simulink model "test"  (R2017b)
settings: Solver=FixedStepDiscrete  StartTime=0.0  StopTime=Inf  FixedStep=Ts  RelTol=1e-3
PreLoadFcn:
  | Ts = 0.01;
PostLoadFcn:
  | , if any(exist('dsrtsu_mdlpostloadfcn', 'file') == [2, 3, 6]), try dsrtsu_mdlpostloadfcn('Execute', bdroot); catch fprintf('Error in PostLoadFcn (dsrtsu_mdlpostloadfcn) for model "%s":\n %s\n', bdroot, lasterr); end, end,
libraries: rtican x19, simulink x9, rti1401lib_adc_type4 x3
(part 5 of 6)

== system test/Hardware ActValue/Suspension Motor RX ==
  N20_TPDO0 : rtican/RTICAN Receive (RX)   Reserved1=[]  Reserved2=[]  Reserved3=[]  Reserved4=[]  SfcnMessage=[]  Msg_Struct=[]  BoardTypeNo=[]  BoardNo=[]  ChannelNo=[]  Parameters=[]  DialogFcn=[]  UnitName=[]  Revision=[]  UnitValues=[]  DSProperties=struct('RTI',struct('Version',uint32(5),'BlockType',struct('isSLSource',uint8(1),'isSLSink',uint8(1),'isHWSource',uint8(0),'isHWSink',uint8(0),'isSetup',uint8(0),'isInline',uint8(1),'isNonInline',uint8(0),'isInterrupt',uint8(0),'isChannelwise',uint8(0)),'IOBoardType','RTICAN','UnitType','MESSAGE','Identifier','RX','DialogType','MSVC','BlockSet','RTICAN','SlaveProcessor','CAN'))  RTIBlockInterface=struct('OutputPortsWidth',int32([1 1 1 1 1 1 1]),'OutputPortsActive',[1 1 1 1 1 1 1],'OutputPortsName',{{'Controlword','Statusword','Modes_of_operation_display','Error_code',['RX status'],['RX time'],['RX delta time']}},'OutputPortsDataType',{{'SS_DOUBLE','SS_DOUBLE','SS_DOUBLE','SS_DOUBLE','SS_DOUBLE','SS_DOUBLE','SS_DOUBLE'}},'OutputPortsLabel',{{'Controlword','Statusword','Modes_of_operation_display','Error_code','','',''}},'OutputPortsLabelMode','ON','InputPortsWidth',int32(0),'InputPortsActive',0,'DialogFcn','rtican_message_interface_gui','BlockDisplay',{{'','center'}},'IconTransparency','on','ParameterTunableNames',{{}},'InitLevel',3,'BlockName',struct('Token',{{'N20_TPDO0'}}),'SampleTime',{{-1}},'TriggerPort',{{'none'}},'EnablePort',{{'none'}})  RTIBlockParameters=struct('BoardTypeNo',{{1,'OFF',[]}},'BoardNo',{{1,'ON',[1 16]}},'ChannelNo',{{1,'ON',[1 2]}},'Parameters',{{struct('DataFileSupport',struct('DataFileSelectedMaster',1,'DataFileSelectedLocal',1,'DataFileName','c:\users\user\desktop\ycm\rcp\can1_canopen.dbc|','DataFileDate',['16-7-2025 15:06:12'],'SelectedFile',['..\..\ycm\rcp\ycm_canopen_v1 .dbc'],'InterfaceFcn','rtican_dbc_file_parser'),'Options',struct('StatusSelected',1,'TimeSelected',1,'DeltaTimeSelected',1,'BytePortSelected',0,'MessageLengthSelected',0,'TriggerPort',struct('Selected',0,'TriggerType',0),'UserCoding',struct('Selected',0,'InterfaceFile','UserDecodingFile','FcnName','UserDecodeFcn','InportSelected',0,'InportWidth',1,'OutportSelected',0,'OutportWidth',1),'EnablePortSelected',0,'SignalOnPortnameSelected',1,'UseRXService',0),'Message',struct('MsgOnBlocknameSelected',1,'MsgName','N20_TPDO0','MsgIdFormat',0,'MsgId',801,'MsgLength',7,'NumSignals',4,'SampleTime',-1,'Signal',struct('SgnName',{'Controlword','Statusword','Modes_of_operation_display','Error_code'},'SgnStartBit',{0,16,32,40},'SgnLength',{16,16,8,16},'ByteLayout',{0,0,0,0},'Factor',{1,1,1,1},'Offset',{0,0,0,0},'SgnComment',{'','','',''},'SgnUnit',{'','','',''},'Min',{0,0,0,0},'Max',{0,0,0,0},'SgnType',{0,0,0,0},'SLDataType',{'SS_DOUBLE','SS_DOUBLE','SS_DOUBLE','SS_DOUBLE'},'DataType',{0,0,1,0},'ModeValue',{-1,-1,-1,-1}),'MsgIdNumFormat',0,'MsgComment',{{''}}),'Version',1.2,'general',struct('isFromLib',0)),'OFF',[]}},'GroupId',{{struct('Group',{{'RTICAN'}},'No',1,'Behavior',{{'NAMECHANGE'}},'BlockType',{{'SINK'}},'NameChangeFlag',0),'OFF',[]}},'SFcnRTICANMessage',{{struct('MsgType','RX','SFcnPortType','Scalar','MsgName','N20_TPDO0','MsgIdFormat','STD','MsgId',801,'MsgLength',7,'NumSignals',4,'SampleTime',-1,'Signal',struct('SgnName',{'Controlword','Statusword','Modes_of_operation_display','Error_code'},'SgnStartBit',{0,16,32,40},'SgnLength',{16,16,8,16},'ByteLayout',{['little endian'],['little endian'],['little endian'],['little endian']},'Factor',{1,1,1,1},'Offset',{0,0,0,0},'SgnType',{'standard','standard','standard','standard'},'SLDataType',{'SS_DOUBLE','SS_DOUBLE','SS_DOUBLE','SS_DOUBLE'},'DataType',{['unsigned int'],['unsigned int'],['signed int'],['unsigned int']},'ModeValue',{-1,-1,-1,-1}),'StatusSelected','yes','TimeSelected','yes','DeltaTimeSelected','yes','BytePortSelected','no','MessageLengthSelected','no','TriggerPort',struct('Selected','no','TriggerType',0),'UserCoding',struct('Selected','no','InterfaceFile','UserDecodingFile','FcnName','UserDecodeFcn','InportSelected','no','InportWidth',1,'OutportSelected','no','OutportWidth',1),'EnablePortSelected','no','UseRXService','no','BoardType','DS1','BoardNo',1,'ControllerNo',1),'OFF',[]}},'TLCFileName',{{'rtican_rx_message','OFF',[]}})  RTISFcnParameters=struct('SFcnRTICANMessage','struct','TLCFileName','char')  RTIBlockParaDefault=struct('BoardTypeNo',4302,'BoardNo',1,'ChannelNo',1,'Parameters',struct('DataFileSupport',struct('DataFileSelectedMaster',0,'DataFileSelectedLocal',0,'DataFileName','','DataFileDate','','SelectedFile',['<no file selected>']),'Options',struct('StatusSelected',1,'TimeSelected',1,'DeltaTimeSelected',1,'BytePortSelected',0,'MessageLengthSelected',0,'TriggerPort',struct('Selected',0,'TriggerType','rising'),'UserCoding',struct('Selected',0,'InterfaceFile','UserDecodingFile','FcnName','UserDecodeFcn','InportSelected',0,'InportWidth',1,'OutportSelected',0,'OutportWidth',1),'EnablePortSelected',0,'SignalOnPortnameSelected',1,'UseRXService',0),'Message',struct('MsgOnBlocknameSelected',0,'MsgName',['RX Message'],'MsgIdFormat',0,'MsgId',100,'MsgLength',8,'NumSignals',1,'SampleTime',-1,'Signal',struct('SgnName',['RX signal'],'SgnStartBit',0,'SgnLength',8,'SgnType',0,'ModeValue',-1,'DataType',0,'SLDataType','SS_DOUBLE','ByteLayout',0,'Factor',1,'Offset',0,'Min',0,'Max',255,'SgnComment',{{}},'SgnUnit',''),'MsgIdNumFormat',0,'MsgComment',{{''}}),'Version',1.2,'general',struct('isFromLib',1)),'GroupId',struct('Group',{{'RTICAN'}},'No',1,'Behavior',{{'NAMECHANGE'}},'BlockType',{{'SINK'}},'NameChangeFlag',0),'SFcnRTICANMessage',struct('MsgType','RX','MsgName',['RX Message'],'MsgIdFormat','STD','MsgId',100,'MsgLength',8,'NumSignals',1,'SampleTime',-1,'Signal',struct('SgnName',['RX signal'],'SgnStartBit',0,'SgnLength',8,'SgnType','standard','ModeValue',-1,'DataType',['unsigned int'],'ByteLayout',['little endian'],'SLDataType','SS_DOUBLE','Factor',1,'Offset',0),'StatusSelected','yes','TimeSelected','yes','DeltaTimeSelected','yes','BytePortSelected','no','MessageLengthSelected','no','EnablePortSelected','no','UserCoding',struct('Selected','no','InterfaceFile','UserDecodingFile','FcnName','UserDecodeFcn','InportSelected','no','InportWidth',1,'OutportSelected','no','OutportWidth',1),'TriggerPort',struct('Selected','no','TriggerType','rising'),'UseRXService','no','BoardType','DS4302','BoardNo',1,'ControllerNo',1,'SFcnPortType','Scalar'),'TLCFileName','rtican_rx_message')
      settings: AttributesFormatString=Group Id: RTICAN1\n  SourceProductName=dSPACE RTI CAN Blockset
  N20_TPDO1 : rtican/RTICAN Receive (RX)   Reserved1=[]  Reserved2=[]  Reserved3=[]  Reserved4=[]  SfcnMessage=[]  Msg_Struct=[]  BoardTypeNo=[]  BoardNo=[]  ChannelNo=[]  Parameters=[]  DialogFcn=[]  UnitName=[]  Revision=[]  UnitValues=[]  DSProperties=struct('RTI',struct('Version',uint32(5),'BlockType',struct('isSLSource',uint8(1),'isSLSink',uint8(1),'isHWSource',uint8(0),'isHWSink',uint8(0),'isSetup',uint8(0),'isInline',uint8(1),'isNonInline',uint8(0),'isInterrupt',uint8(0),'isChannelwise',uint8(0)),'IOBoardType','RTICAN','UnitType','MESSAGE','Identifier','RX','DialogType','MSVC','BlockSet','RTICAN','SlaveProcessor','CAN'))  RTIBlockInterface=struct('OutputPortsWidth',int32([1 1 1 1 1]),'OutputPortsActive',[1 1 1 1 1],'OutputPortsName',{{'Position_demand_value','Position_actual_value',['RX status'],['RX time'],['RX delta time']}},'OutputPortsDataType',{{'SS_DOUBLE','SS_DOUBLE','SS_DOUBLE','SS_DOUBLE','SS_DOUBLE'}},'OutputPortsLabel',{{'Position_demand_value','Position_actual_value','','',''}},'OutputPortsLabelMode','ON','InputPortsWidth',int32(0),'InputPortsActive',0,'DialogFcn','rtican_message_interface_gui','BlockDisplay',{{'','center'}},'IconTransparency','on','ParameterTunableNames',{{}},'InitLevel',3,'BlockName',struct('Token',{{'N20_TPDO1'}}),'SampleTime',{{-1}},'TriggerPort',{{'none'}},'EnablePort',{{'none'}})  RTIBlockParameters=struct('BoardTypeNo',{{1,'OFF',[]}},'BoardNo',{{1,'ON',[1 16]}},'ChannelNo',{{1,'ON',[1 2]}},'Parameters',{{struct('DataFileSupport',struct('DataFileSelectedMaster',1,'DataFileSelectedLocal',1,'DataFileName','c:\users\user\desktop\ycm\rcp\can1_canopen.dbc|','DataFileDate',['16-7-2025 15:06:12'],'SelectedFile',['..\..\ycm\rcp\ycm_canopen_v1 .dbc'],'InterfaceFcn','rtican_dbc_file_parser'),'Options',struct('StatusSelected',1,'TimeSelected',1,'DeltaTimeSelected',1,'BytePortSelected',0,'MessageLengthSelected',0,'TriggerPort',struct('Selected',0,'TriggerType',0),'UserCoding',struct('Selected',0,'InterfaceFile','UserDecodingFile','FcnName','UserDecodeFcn','InportSelected',0,'InportWidth',1,'OutportSelected',0,'OutportWidth',1),'EnablePortSelected',0,'SignalOnPortnameSelected',1,'UseRXService',0),'Message',struct('MsgOnBlocknameSelected',1,'MsgName','N20_TPDO1','MsgIdFormat',0,'MsgId',802,'MsgLength',8,'NumSignals',2,'SampleTime',-1,'Signal',struct('SgnName',{'Position_demand_value','Position_actual_value'},'SgnStartBit',{0,32},'SgnLength',{32,32},'ByteLayout',{0,0},'Factor',{1,1},'Offset',{0,0},'SgnComment',{'',''},'SgnUnit',{'',''},'Min',{0,0},'Max',{0,0},'SgnType',{0,0},'SLDataType',{'SS_DOUBLE','SS_DOUBLE'},'DataType',{1,1},'ModeValue',{-1,-1}),'MsgIdNumFormat',0,'MsgComment',{{''}}),'Version',1.2,'general',struct('isFromLib',0)),'OFF',[]}},'GroupId',{{struct('Group',{{'RTICAN'}},'No',1,'Behavior',{{'NAMECHANGE'}},'BlockType',{{'SINK'}},'NameChangeFlag',0),'OFF',[]}},'SFcnRTICANMessage',{{struct('MsgType','RX','SFcnPortType','Scalar','MsgName','N20_TPDO1','MsgIdFormat','STD','MsgId',802,'MsgLength',8,'NumSignals',2,'SampleTime',-1,'Signal',struct('SgnName',{'Position_demand_value','Position_actual_value'},'SgnStartBit',{0,32},'SgnLength',{32,32},'ByteLayout',{['little endian'],['little endian']},'Factor',{1,1},'Offset',{0,0},'SgnType',{'standard','standard'},'SLDataType',{'SS_DOUBLE','SS_DOUBLE'},'DataType',{['signed int'],['signed int']},'ModeValue',{-1,-1}),'StatusSelected','yes','TimeSelected','yes','DeltaTimeSelected','yes','BytePortSelected','no','MessageLengthSelected','no','TriggerPort',struct('Selected','no','TriggerType',0),'UserCoding',struct('Selected','no','InterfaceFile','UserDecodingFile','FcnName','UserDecodeFcn','InportSelected','no','InportWidth',1,'OutportSelected','no','OutportWidth',1),'EnablePortSelected','no','UseRXService','no','BoardType','DS1','BoardNo',1,'ControllerNo',1),'OFF',[]}},'TLCFileName',{{'rtican_rx_message','OFF',[]}})  RTISFcnParameters=struct('SFcnRTICANMessage','struct','TLCFileName','char')  RTIBlockParaDefault=struct('BoardTypeNo',4302,'BoardNo',1,'ChannelNo',1,'Parameters',struct('DataFileSupport',struct('DataFileSelectedMaster',0,'DataFileSelectedLocal',0,'DataFileName','','DataFileDate','','SelectedFile',['<no file selected>']),'Options',struct('StatusSelected',1,'TimeSelected',1,'DeltaTimeSelected',1,'BytePortSelected',0,'MessageLengthSelected',0,'TriggerPort',struct('Selected',0,'TriggerType','rising'),'UserCoding',struct('Selected',0,'InterfaceFile','UserDecodingFile','FcnName','UserDecodeFcn','InportSelected',0,'InportWidth',1,'OutportSelected',0,'OutportWidth',1),'EnablePortSelected',0,'SignalOnPortnameSelected',1,'UseRXService',0),'Message',struct('MsgOnBlocknameSelected',0,'MsgName',['RX Message'],'MsgIdFormat',0,'MsgId',100,'MsgLength',8,'NumSignals',1,'SampleTime',-1,'Signal',struct('SgnName',['RX signal'],'SgnStartBit',0,'SgnLength',8,'SgnType',0,'ModeValue',-1,'DataType',0,'SLDataType','SS_DOUBLE','ByteLayout',0,'Factor',1,'Offset',0,'Min',0,'Max',255,'SgnComment',{{}},'SgnUnit',''),'MsgIdNumFormat',0,'MsgComment',{{''}}),'Version',1.2,'general',struct('isFromLib',1)),'GroupId',struct('Group',{{'RTICAN'}},'No',1,'Behavior',{{'NAMECHANGE'}},'BlockType',{{'SINK'}},'NameChangeFlag',0),'SFcnRTICANMessage',struct('MsgType','RX','MsgName',['RX Message'],'MsgIdFormat','STD','MsgId',100,'MsgLength',8,'NumSignals',1,'SampleTime',-1,'Signal',struct('SgnName',['RX signal'],'SgnStartBit',0,'SgnLength',8,'SgnType','standard','ModeValue',-1,'DataType',['unsigned int'],'ByteLayout',['little endian'],'SLDataType','SS_DOUBLE','Factor',1,'Offset',0),'StatusSelected','yes','TimeSelected','yes','DeltaTimeSelected','yes','BytePortSelected','no','MessageLengthSelected','no','EnablePortSelected','no','UserCoding',struct('Selected','no','InterfaceFile','UserDecodingFile','FcnName','UserDecodeFcn','InportSelected','no','InportWidth',1,'OutportSelected','no','OutportWidth',1),'TriggerPort',struct('Selected','no','TriggerType','rising'),'UseRXService','no','BoardType','DS4302','BoardNo',1,'ControllerNo',1,'SFcnPortType','Scalar'),'TLCFileName','rtican_rx_message')
      settings: AttributesFormatString=Group Id: RTICAN1\n  SourceProductName=dSPACE RTI CAN Blockset
  N20_TPDO2 : rtican/RTICAN Receive (RX)   Reserved1=[]  Reserved2=[]  Reserved3=[]  Reserved4=[]  SfcnMessage=[]  Msg_Struct=[]  BoardTypeNo=[]  BoardNo=[]  ChannelNo=[]  Parameters=[]  DialogFcn=[]  UnitName=[]  Revision=[]  UnitValues=[]  DSProperties=struct('RTI',struct('Version',uint32(5),'BlockType',struct('isSLSource',uint8(1),'isSLSink',uint8(1),'isHWSource',uint8(0),'isHWSink',uint8(0),'isSetup',uint8(0),'isInline',uint8(1),'isNonInline',uint8(0),'isInterrupt',uint8(0),'isChannelwise',uint8(0)),'IOBoardType','RTICAN','UnitType','MESSAGE','Identifier','RX','DialogType','MSVC','BlockSet','RTICAN','SlaveProcessor','CAN'))  RTIBlockInterface=struct('OutputPortsWidth',int32([1 1 1 1 1]),'OutputPortsActive',[1 1 1 1 1],'OutputPortsName',{{'Velocity_demand_value','Velocity_actual_value_averaged',['RX status'],['RX time'],['RX delta time']}},'OutputPortsDataType',{{'SS_DOUBLE','SS_DOUBLE','SS_DOUBLE','SS_DOUBLE','SS_DOUBLE'}},'OutputPortsLabel',{{'Velocity_demand_value','Velocity_actual_value_averaged','','',''}},'OutputPortsLabelMode','ON','InputPortsWidth',int32(0),'InputPortsActive',0,'DialogFcn','rtican_message_interface_gui','BlockDisplay',{{'','center'}},'IconTransparency','on','ParameterTunableNames',{{}},'InitLevel',3,'BlockName',struct('Token',{{'N20_TPDO2'}}),'SampleTime',{{-1}},'TriggerPort',{{'none'}},'EnablePort',{{'none'}})  RTIBlockParameters=struct('BoardTypeNo',{{1,'OFF',[]}},'BoardNo',{{1,'ON',[1 16]}},'ChannelNo',{{1,'ON',[1 2]}},'Parameters',{{struct('DataFileSupport',struct('DataFileSelectedMaster',1,'DataFileSelectedLocal',1,'DataFileName','c:\users\user\desktop\ycm\rcp\can1_canopen.dbc|','DataFileDate',['16-7-2025 15:06:12'],'SelectedFile',['..\..\ycm\rcp\ycm_canopen_v1 .dbc'],'InterfaceFcn','rtican_dbc_file_parser'),'Options',struct('StatusSelected',1,'TimeSelected',1,'DeltaTimeSelected',1,'BytePortSelected',0,'MessageLengthSelected',0,'TriggerPort',struct('Selected',0,'TriggerType',0),'UserCoding',struct('Selected',0,'InterfaceFile','UserDecodingFile','FcnName','UserDecodeFcn','InportSelected',0,'InportWidth',1,'OutportSelected',0,'OutportWidth',1),'EnablePortSelected',0,'SignalOnPortnameSelected',1,'UseRXService',0),'Message',struct('MsgOnBlocknameSelected',1,'MsgName','N20_TPDO2','MsgIdFormat',0,'MsgId',803,'MsgLength',8,'NumSignals',2,'SampleTime',-1,'Signal',struct('SgnName',{'Velocity_demand_value','Velocity_actual_value_averaged'},'SgnStartBit',{0,32},'SgnLength',{32,32},'ByteLayout',{0,0},'Factor',{1,1},'Offset',{0,0},'SgnComment',{'',''},'SgnUnit',{'',''},'Min',{0,0},'Max',{0,0},'SgnType',{0,0},'SLDataType',{'SS_DOUBLE','SS_DOUBLE'},'DataType',{1,1},'ModeValue',{-1,-1}),'MsgIdNumFormat',0,'MsgComment',{{''}}),'Version',1.2,'general',struct('isFromLib',0)),'OFF',[]}},'GroupId',{{struct('Group',{{'RTICAN'}},'No',1,'Behavior',{{'NAMECHANGE'}},'BlockType',{{'SINK'}},'NameChangeFlag',0),'OFF',[]}},'SFcnRTICANMessage',{{struct('MsgType','RX','SFcnPortType','Scalar','MsgName','N20_TPDO2','MsgIdFormat','STD','MsgId',803,'MsgLength',8,'NumSignals',2,'SampleTime',-1,'Signal',struct('SgnName',{'Velocity_demand_value','Velocity_actual_value_averaged'},'SgnStartBit',{0,32},'SgnLength',{32,32},'ByteLayout',{['little endian'],['little endian']},'Factor',{1,1},'Offset',{0,0},'SgnType',{'standard','standard'},'SLDataType',{'SS_DOUBLE','SS_DOUBLE'},'DataType',{['signed int'],['signed int']},'ModeValue',{-1,-1}),'StatusSelected','yes','TimeSelected','yes','DeltaTimeSelected','yes','BytePortSelected','no','MessageLengthSelected','no','TriggerPort',struct('Selected','no','TriggerType',0),'UserCoding',struct('Selected','no','InterfaceFile','UserDecodingFile','FcnName','UserDecodeFcn','InportSelected','no','InportWidth',1,'OutportSelected','no','OutportWidth',1),'EnablePortSelected','no','UseRXService','no','BoardType','DS1','BoardNo',1,'ControllerNo',1),'OFF',[]}},'TLCFileName',{{'rtican_rx_message','OFF',[]}})  RTISFcnParameters=struct('SFcnRTICANMessage','struct','TLCFileName','char')  RTIBlockParaDefault=struct('BoardTypeNo',4302,'BoardNo',1,'ChannelNo',1,'Parameters',struct('DataFileSupport',struct('DataFileSelectedMaster',0,'DataFileSelectedLocal',0,'DataFileName','','DataFileDate','','SelectedFile',['<no file selected>']),'Options',struct('StatusSelected',1,'TimeSelected',1,'DeltaTimeSelected',1,'BytePortSelected',0,'MessageLengthSelected',0,'TriggerPort',struct('Selected',0,'TriggerType','rising'),'UserCoding',struct('Selected',0,'InterfaceFile','UserDecodingFile','FcnName','UserDecodeFcn','InportSelected',0,'InportWidth',1,'OutportSelected',0,'OutportWidth',1),'EnablePortSelected',0,'SignalOnPortnameSelected',1,'UseRXService',0),'Message',struct('MsgOnBlocknameSelected',0,'MsgName',['RX Message'],'MsgIdFormat',0,'MsgId',100,'MsgLength',8,'NumSignals',1,'SampleTime',-1,'Signal',struct('SgnName',['RX signal'],'SgnStartBit',0,'SgnLength',8,'SgnType',0,'ModeValue',-1,'DataType',0,'SLDataType','SS_DOUBLE','ByteLayout',0,'Factor',1,'Offset',0,'Min',0,'Max',255,'SgnComment',{{}},'SgnUnit',''),'MsgIdNumFormat',0,'MsgComment',{{''}}),'Version',1.2,'general',struct('isFromLib',1)),'GroupId',struct('Group',{{'RTICAN'}},'No',1,'Behavior',{{'NAMECHANGE'}},'BlockType',{{'SINK'}},'NameChangeFlag',0),'SFcnRTICANMessage',struct('MsgType','RX','MsgName',['RX Message'],'MsgIdFormat','STD','MsgId',100,'MsgLength',8,'NumSignals',1,'SampleTime',-1,'Signal',struct('SgnName',['RX signal'],'SgnStartBit',0,'SgnLength',8,'SgnType','standard','ModeValue',-1,'DataType',['unsigned int'],'ByteLayout',['little endian'],'SLDataType','SS_DOUBLE','Factor',1,'Offset',0),'StatusSelected','yes','TimeSelected','yes','DeltaTimeSelected','yes','BytePortSelected','no','MessageLengthSelected','no','EnablePortSelected','no','UserCoding',struct('Selected','no','InterfaceFile','UserDecodingFile','FcnName','UserDecodeFcn','InportSelected','no','InportWidth',1,'OutportSelected','no','OutportWidth',1),'TriggerPort',struct('Selected','no','TriggerType','rising'),'UseRXService','no','BoardType','DS4302','BoardNo',1,'ControllerNo',1,'SFcnPortType','Scalar'),'TLCFileName','rtican_rx_message')
      settings: AttributesFormatString=Group Id: RTICAN1\n  SourceProductName=dSPACE RTI CAN Blockset
  N20_TPDO3 : rtican/RTICAN Receive (RX)   Reserved1=[]  Reserved2=[]  Reserved3=[]  Reserved4=[]  SfcnMessage=[]  Msg_Struct=[]  BoardTypeNo=[]  BoardNo=[]  ChannelNo=[]  Parameters=[]  DialogFcn=[]  UnitName=[]  Revision=[]  UnitValues=[]  DSProperties=struct('RTI',struct('Version',uint32(5),'BlockType',struct('isSLSource',uint8(1),'isSLSink',uint8(1),'isHWSource',uint8(0),'isHWSink',uint8(0),'isSetup',uint8(0),'isInline',uint8(1),'isNonInline',uint8(0),'isInterrupt',uint8(0),'isChannelwise',uint8(0)),'IOBoardType','RTICAN','UnitType','MESSAGE','Identifier','RX','DialogType','MSVC','BlockSet','RTICAN','SlaveProcessor','CAN'))  RTIBlockInterface=struct('OutputPortsWidth',int32([1 1 1 1 1]),'OutputPortsActive',[1 1 1 1 1],'OutputPortsName',{{'Current_demand_value','Current_actual_value_averaged',['RX status'],['RX time'],['RX delta time']}},'OutputPortsDataType',{{'SS_DOUBLE','SS_DOUBLE','SS_DOUBLE','SS_DOUBLE','SS_DOUBLE'}},'OutputPortsLabel',{{'Current_demand_value','Current_actual_value_averaged','','',''}},'OutputPortsLabelMode','ON','InputPortsWidth',int32(0),'InputPortsActive',0,'DialogFcn','rtican_message_interface_gui','BlockDisplay',{{'','center'}},'IconTransparency','on','ParameterTunableNames',{{}},'InitLevel',3,'BlockName',struct('Token',{{'N20_TPDO3'}}),'SampleTime',{{-1}},'TriggerPort',{{'none'}},'EnablePort',{{'none'}})  RTIBlockParameters=struct('BoardTypeNo',{{1,'OFF',[]}},'BoardNo',{{1,'ON',[1 16]}},'ChannelNo',{{1,'ON',[1 2]}},'Parameters',{{struct('DataFileSupport',struct('DataFileSelectedMaster',1,'DataFileSelectedLocal',1,'DataFileName','c:\users\user\desktop\ycm\rcp\can1_canopen.dbc|','DataFileDate',['16-7-2025 15:06:12'],'SelectedFile',['..\..\ycm\rcp\ycm_canopen_v1 .dbc'],'InterfaceFcn','rtican_dbc_file_parser'),'Options',struct('StatusSelected',1,'TimeSelected',1,'DeltaTimeSelected',1,'BytePortSelected',0,'MessageLengthSelected',0,'TriggerPort',struct('Selected',0,'TriggerType',0),'UserCoding',struct('Selected',0,'InterfaceFile','UserDecodingFile','FcnName','UserDecodeFcn','InportSelected',0,'InportWidth',1,'OutportSelected',0,'OutportWidth',1),'EnablePortSelected',0,'SignalOnPortnameSelected',1,'UseRXService',0),'Message',struct('MsgOnBlocknameSelected',1,'MsgName','N20_TPDO3','MsgIdFormat',0,'MsgId',804,'MsgLength',8,'NumSignals',2,'SampleTime',-1,'Signal',struct('SgnName',{'Current_demand_value','Current_actual_value_averaged'},'SgnStartBit',{0,32},'SgnLength',{32,32},'ByteLayout',{0,0},'Factor',{1,1},'Offset',{0,0},'SgnComment',{'',''},'SgnUnit',{'',''},'Min',{0,0},'Max',{0,0},'SgnType',{0,0},'SLDataType',{'SS_DOUBLE','SS_DOUBLE'},'DataType',{1,1},'ModeValue',{-1,-1}),'MsgIdNumFormat',0,'MsgComment',{{''}}),'Version',1.2,'general',struct('isFromLib',0)),'OFF',[]}},'GroupId',{{struct('Group',{{'RTICAN'}},'No',1,'Behavior',{{'NAMECHANGE'}},'BlockType',{{'SINK'}},'NameChangeFlag',0),'OFF',[]}},'SFcnRTICANMessage',{{struct('MsgType','RX','SFcnPortType','Scalar','MsgName','N20_TPDO3','MsgIdFormat','STD','MsgId',804,'MsgLength',8,'NumSignals',2,'SampleTime',-1,'Signal',struct('SgnName',{'Current_demand_value','Current_actual_value_averaged'},'SgnStartBit',{0,32},'SgnLength',{32,32},'ByteLayout',{['little endian'],['little endian']},'Factor',{1,1},'Offset',{0,0},'SgnType',{'standard','standard'},'SLDataType',{'SS_DOUBLE','SS_DOUBLE'},'DataType',{['signed int'],['signed int']},'ModeValue',{-1,-1}),'StatusSelected','yes','TimeSelected','yes','DeltaTimeSelected','yes','BytePortSelected','no','MessageLengthSelected','no','TriggerPort',struct('Selected','no','TriggerType',0),'UserCoding',struct('Selected','no','InterfaceFile','UserDecodingFile','FcnName','UserDecodeFcn','InportSelected','no','InportWidth',1,'OutportSelected','no','OutportWidth',1),'EnablePortSelected','no','UseRXService','no','BoardType','DS1','BoardNo',1,'ControllerNo',1),'OFF',[]}},'TLCFileName',{{'rtican_rx_message','OFF',[]}})  RTISFcnParameters=struct('SFcnRTICANMessage','struct','TLCFileName','char')  RTIBlockParaDefault=struct('BoardTypeNo',4302,'BoardNo',1,'ChannelNo',1,'Parameters',struct('DataFileSupport',struct('DataFileSelectedMaster',0,'DataFileSelectedLocal',0,'DataFileName','','DataFileDate','','SelectedFile',['<no file selected>']),'Options',struct('StatusSelected',1,'TimeSelected',1,'DeltaTimeSelected',1,'BytePortSelected',0,'MessageLengthSelected',0,'TriggerPort',struct('Selected',0,'TriggerType','rising'),'UserCoding',struct('Selected',0,'InterfaceFile','UserDecodingFile','FcnName','UserDecodeFcn','InportSelected',0,'InportWidth',1,'OutportSelected',0,'OutportWidth',1),'EnablePortSelected',0,'SignalOnPortnameSelected',1,'UseRXService',0),'Message',struct('MsgOnBlocknameSelected',0,'MsgName',['RX Message'],'MsgIdFormat',0,'MsgId',100,'MsgLength',8,'NumSignals',1,'SampleTime',-1,'Signal',struct('SgnName',['RX signal'],'SgnStartBit',0,'SgnLength',8,'SgnType',0,'ModeValue',-1,'DataType',0,'SLDataType','SS_DOUBLE','ByteLayout',0,'Factor',1,'Offset',0,'Min',0,'Max',255,'SgnComment',{{}},'SgnUnit',''),'MsgIdNumFormat',0,'MsgComment',{{''}}),'Version',1.2,'general',struct('isFromLib',1)),'GroupId',struct('Group',{{'RTICAN'}},'No',1,'Behavior',{{'NAMECHANGE'}},'BlockType',{{'SINK'}},'NameChangeFlag',0),'SFcnRTICANMessage',struct('MsgType','RX','MsgName',['RX Message'],'MsgIdFormat','STD','MsgId',100,'MsgLength',8,'NumSignals',1,'SampleTime',-1,'Signal',struct('SgnName',['RX signal'],'SgnStartBit',0,'SgnLength',8,'SgnType','standard','ModeValue',-1,'DataType',['unsigned int'],'ByteLayout',['little endian'],'SLDataType','SS_DOUBLE','Factor',1,'Offset',0),'StatusSelected','yes','TimeSelected','yes','DeltaTimeSelected','yes','BytePortSelected','no','MessageLengthSelected','no','EnablePortSelected','no','UserCoding',struct('Selected','no','InterfaceFile','UserDecodingFile','FcnName','UserDecodeFcn','InportSelected','no','InportWidth',1,'OutportSelected','no','OutportWidth',1),'TriggerPort',struct('Selected','no','TriggerType','rising'),'UseRXService','no','BoardType','DS4302','BoardNo',1,'ControllerNo',1,'SFcnPortType','Scalar'),'TLCFileName','rtican_rx_message')
      settings: AttributesFormatString=Group Id: RTICAN1\n  SourceProductName=dSPACE RTI CAN Blockset
  Controlword : Outport
  Statusword : Outport  Port=2
  Modes_of_operation_display : Outport  Port=3
  Error_code : Outport  Port=4
  Position_demand_value : Outport  Port=5
  Position_actual_value : Outport  Port=6
  Velocity_demand_value : Outport  Port=7
  Velocity_actual_value_averaged : Outport  Port=8
  Current_demand_value : Outport  Port=9
  Current_actual_value_averaged : Outport  Port=10
  wires:
  N20_TPDO2/2 -> Velocity_actual_value_averaged/1  "Velocity_actual_value_averaged"
  N20_TPDO2/1 -> Velocity_demand_value/1  "Velocity_demand_value"
  N20_TPDO0/1 -> Controlword/1  "Controlword"
  N20_TPDO1/2 -> Position_actual_value/1  "Position_actual_value"
  N20_TPDO0/2 -> Statusword/1  "Statusword"
  N20_TPDO1/1 -> Position_demand_value/1  "Position_demand_value"
  N20_TPDO0/3 -> Modes_of_operation_display/1  "Modes_of_operation_display"
  N20_TPDO0/4 -> Error_code/1  "Error_code"
  N20_TPDO3/1 -> Current_demand_value/1  "Current_demand_value"
  N20_TPDO3/2 -> Current_actual_value_averaged/1  "Current_actual_value_averaged"

== system test/RTI Data/RTI Data Store ==
  RTI Data Store : Subsystem  mask(RTI_DATA_STORE){}
      mask help:
      | RTI Data Store Block. This block is used by RTI to store internal model dependent data. Deleting this block will result in data loss.
      |
      | NEVER DELETE, COPY, OR MODIFY THIS BLOCK!
      mask Help:
      | RTI Data Store Block. This block is used by RTI to store internal model dependent data. Deleting this block will result in data loss.
      | 
      | NEVER DELETE, COPY, OR MODIFY THIS BLOCK!
      mask Display: text(0.5, 0.5, ' ', 'HorizontalAlignment', 'center');

== system test/_Reference/_ID_ref ==
  note: Driving Motor Rated Torque: 55.08 mNm
  note: mN*m
  note: A
  note: Steering Motor Rated Torque: 55.08 mNm
  Add : Sum
  Constant : Constant  Value=55.08
  Constant1 : Constant
  Constant2 : Constant  Value=0
  Constant3 : Constant
  Divide : Product  Inputs=*/
  Divide1 : Product  Inputs=**
  Divide2 : Product  Inputs=**
  From Workspace : FromWorkspace  VariableName=u_total  SampleTime=0
  Gain : Gain  Gain=1000
  Gain1 : Gain  Gain=1/Ts
  Selector : Selector  NumberOfDimensions=2  InputPortWidth=3  IndexOptions=Index vector (dialog),Index vector (port)  Indices=1,1  OutputSizes=1,1
  Switch : Switch  Criteria=u2 > Threshold  Threshold=120
  Torque Constant : Gain  Gain=51
  tag scope: ID_Target_Torque=global, ID_idx=global, closed_ID_FF=global
  wires:
  Torque Constant/1 -> [closed_ID_FF], Divide/1
  Constant/1 -> Divide/2
  Divide/1 -> Gain/1
  Gain/1 -> [ID_Target_Torque]
  Selector/1 -> Divide1/1
  Constant1/1 -> Add/2
  [ID_idx_Time] -> Gain1/1
  Gain1/1 -> Add/1
  Add/1 -> [ID_idx], Selector/2
  [ID_idx_Time] -> Switch/2
  Constant2/1 -> Switch/1
  Constant3/1 -> Switch/3
  Switch/1 -> Divide1/2
  Divide1/1 -> Divide2/1
  [ID_OnOff] -> Divide2/2
  Divide2/1 -> Torque Constant/1
  From Workspace/1 -> Selector/1

== system test/_Reference/_dri_motor_ref ==
  Constant : Constant  Value=0
  Driving_Torque_Ref : Subsystem
      mask Display: disp('Driving Torque Ref')
  Driving_Vel_Ref : Subsystem
      mask Display: disp('Driving Vel Ref')
  If Action Subsystem1 : Subsystem  TreatAsAtomicUnit=on
  If Action Subsystem2 : Subsystem  TreatAsAtomicUnit=on
  If Action Subsystem3 : Subsystem  TreatAsAtomicUnit=on
  If1 : If  IfExpression=u1 == 9  ElseIfExpressions=u1 == 10
  Merge1 : Merge  Inputs=3
  tag scope: dri_target_vel=global
  wires:
  Merge1/1 -> [dri_target_vel]
  [Mode_of_operation_Ref] -> If1/1
  If1/1 -> If Action Subsystem2/Action
  [dri_velocity_ref_vel] -> If Action Subsystem2/1(In1)
  If1/2 -> If Action Subsystem1/Action
  [dri_torque_ref_vel] -> If Action Subsystem1/1(In1)
  If Action Subsystem2/1(Out1) -> Merge1/1
  If Action Subsystem1/1(Out1) -> Merge1/2
  If1/3 -> If Action Subsystem3/Action
  Constant/1 -> If Action Subsystem3/1(In1)
  If Action Subsystem3/1(Out1) -> Merge1/3

== system test/_Reference/_str_motor_ref ==
  note: Load deg
  note: cnt
  note: Motor deg
  Constant : Constant  Value=360
  Data Type Conversion : DataTypeConversion
  Gain : Gain  Gain=-1
  LPF1 : Subsystem
  Product : Product
  Product1 : Product
  Product2 : Product  Inputs=*/
  Product3 : Product
  Rate Limiter Dynamic : simulink/Discontinuities/Rate Limiter Dynamic
      settings: SourceProductName=Simulink
  Round : Rounding  Operator=round
  Saturation : Saturate  UpperLimit=20  LowerLimit=-20
  Str_Target_pos : Constant  Value=0
  tag scope: str_load_target_pos=global, str_target_pos=global
  wires:
  Product2/1 -> Product1/2
  LPF1/1(Out) -> [str_load_target_pos], Product/1
  [N_str] -> Product/2
  Product/1 -> Product1/1
  [cpt_str] -> Product2/1
  [str_pos_ref_cutoff] -> LPF1/2(fc)
  Constant/1 -> Product2/2
  Product1/1 -> Round/1
  Round/1 -> Data Type Conversion/1
  Data Type Conversion/1 -> [str_target_pos]
  Product3/1 -> Saturation/1
  [ctrl_onoff] -> Product3/1
  Str_Target_pos/1 -> Product3/2
  Saturation/1 -> Rate Limiter Dynamic/2
  Rate Limiter Dynamic/1 -> LPF1/1(In)
  [str_pos_ref_ratelimit] -> Rate Limiter Dynamic/1, Gain/1
  Gain/1 -> Rate Limiter Dynamic/3

== system test/_Reference/_sus_motor_ref ==
  note: cnt
  note: deg
  Constant1 : Constant  Value=360
  Data Type Conversion1 : DataTypeConversion
  Gain : Gain  Gain=-1
  LPF2 : Subsystem
  Product1 : Product
  Product3 : Product
  Product4 : Product
  Product5 : Product  Inputs=*/
  Rate Limiter Dynamic : simulink/Discontinuities/Rate Limiter Dynamic
      settings: SourceProductName=Simulink
  Round1 : Rounding  Operator=round
  Saturation1 : Saturate  UpperLimit=20  LowerLimit=-20
  Sus_Target_pos : Constant  Value=0
  tag scope: sus_target_pos=global
  wires:
  Saturation1/1 -> Rate Limiter Dynamic/2
  [sus_pos_ref_cutoff] -> LPF2/2(fc)
  Round1/1 -> Data Type Conversion1/1
  LPF2/1(Out) -> Product3/1
  [cpt_sus] -> Product5/1
  Rate Limiter Dynamic/1 -> LPF2/1(In)
  Product3/1 -> Product4/1
  Constant1/1 -> Product5/2
  Product4/1 -> Round1/1
  Data Type Conversion1/1 -> [sus_target_pos]
  [N_sus] -> Product3/2
  Product5/1 -> Product4/2
  [ctrl_onoff] -> Product1/1
  Product1/1 -> Saturation1/1
  Sus_Target_pos/1 -> Product1/2
  [sus_pos_ref_ratelimit] -> Gain/1, Rate Limiter Dynamic/1
  Gain/1 -> Rate Limiter Dynamic/3

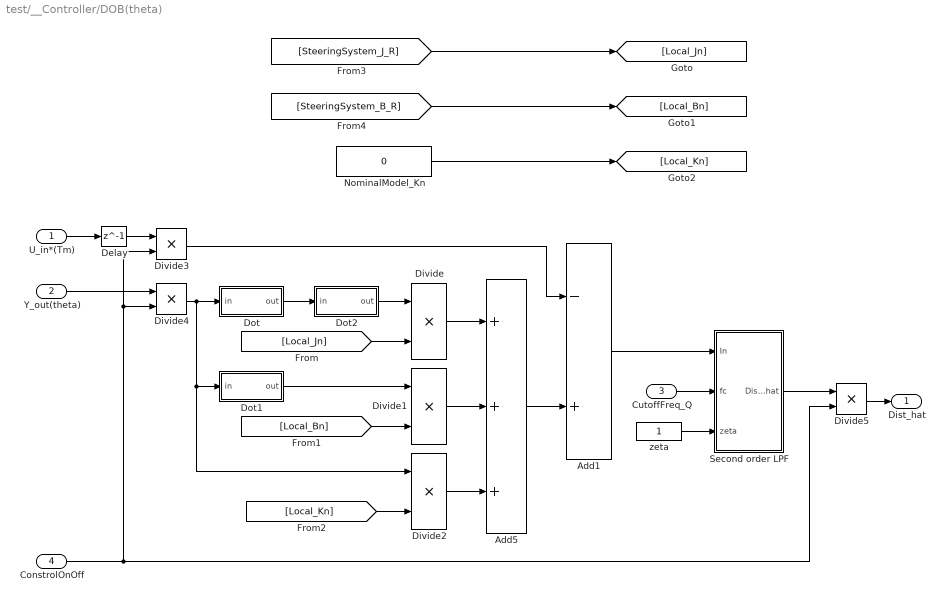
== system test/__Controller/DOB(theta) ==
  U_in*(Tm) : Inport
  Y_out(theta) : Inport  Port=2
  CutoffFreq_Q : Inport  Port=3
  ConstrolOnOff : Inport  Port=4
  Add1 : Sum  Inputs=-+
  Add5 : Sum  Inputs=+++
  Delay : Delay  DelayLength=1  InitialCondition=0
  Divide{,1..5} (6 alike) : Product  Inputs=**
  Dot : Subsystem
      mask Display: disp('dot')
  Dot1 : Subsystem
      mask Display: disp('dot')
  Dot2 : Subsystem
      mask Display: disp('dot')
  NominalModel_Kn : Constant  Value=0
  Second order LPF : Subsystem
  zeta : Constant  SampleTime=Ts
  Dist_hat : Outport
  wires:
  Add1/1 -> Second order LPF/1(In)
  Add5/1 -> Add1/2
  CutoffFreq_Q/1 -> Second order LPF/2(fc)
  zeta/1 -> Second order LPF/3(zeta)
  [SteeringSystem_J_R] -> [Local_Jn]
  NominalModel_Kn/1 -> [Local_Kn]
  [SteeringSystem_B_R] -> [Local_Bn]
  Y_out(theta)/1 -> Divide4/1
  [Local_Jn] -> Divide/2
  [Local_Kn] -> Divide2/2
  Dot1/1(out) -> Divide1/1
  [Local_Bn] -> Divide1/2
  Dot/1(out) -> Dot2/1(in)
  Divide/1 -> Add5/1
  Divide2/1 -> Add5/3
  Divide1/1 -> Add5/2
  Dot2/1(out) -> Divide/1
  ConstrolOnOff/1 -> Divide5/2, Divide3/2, Divide4/2
  Divide4/1 -> Divide2/1, Dot1/1(in), Dot/1(in)
  U_in*(Tm)/1 -> Delay/1
  Divide3/1 -> Add1/1
  Second order LPF/1(Dist_hat) -> Divide5/1
  Divide5/1 -> Dist_hat/1
  Delay/1 -> Divide3/1

== system test/__Controller/Driving Wheel Control ==
  note: okay
  note: okay
  note: okay
  Add : Sum  Inputs=++-
  Add1 : Sum  Inputs=+-
  Constant : Constant  Value=0
  DOB(omega) : Subsystem
  Feedforward(omega) : Subsystem
  Poleplacement(PI)1 : Subsystem
  Subsystem : Subsystem
  tag scope: dri_ctrl_FF=global, dri_ctrl_PID=global, dri_ctrl_Total=global, dri_ctrl_dhat=global, dri_ctrl_torque=global
  wires:
  [dri_target_vel] -> Add1/1, Feedforward(omega)/1(command)
  [dri_ff_cutoff] -> Feedforward(omega)/2(LFP cutoff)
  Subsystem/1(Target Torque) -> [dri_ctrl_torque]
  Feedforward(omega)/1(FF) -> [dri_ctrl_FF], Add/1
  Poleplacement(PI)1/1(feedback gain) -> [dri_ctrl_PID], Add/2
  [Sensor_wheel_angvel] -> DOB(omega)/2(Y_out(w))
  DOB(omega)/1(Dist_hat) -> [dri_ctrl_dhat], Add/3
  Add/1 -> DOB(omega)/1(U_in*(Tm)), [dri_ctrl_Total], Subsystem/1(N*m)
  [dri_ff_onoff] -> Feedforward(omega)/3(ControlOnOff)
  [dri_dob_onoff] -> DOB(omega)/4(ControlOnOff)
  [dri_dob_cutoff] -> DOB(omega)/3(CutoffFreq_Q)
  [dri_pid_zeta] -> Poleplacement(PI)1/3(zeta)
  [Sensor_wheel_angvel] -> Add1/2
  Add1/1 -> Poleplacement(PI)1/1(error)
  [dri_pid_cutoff] -> Poleplacement(PI)1/2(BW)
  [dri_pid_onoff] -> Poleplacement(PI)1/4(ConstrolOnOff)
  Constant/1 -> Poleplacement(PI)1/5(ControlInputError)

== system test/__Controller/If Action Subsystem ==
  In1 : Inport
  Action Port : ActionPort  ActionType=then
  Out1 : Outport
  wires:
  In1/1 -> Out1/1

== system test/__Controller/If Action Subsystem1 ==
  In1 : Inport
  Action Port : ActionPort  ActionType=else
  Out1 : Outport
  wires:
  In1/1 -> Out1/1

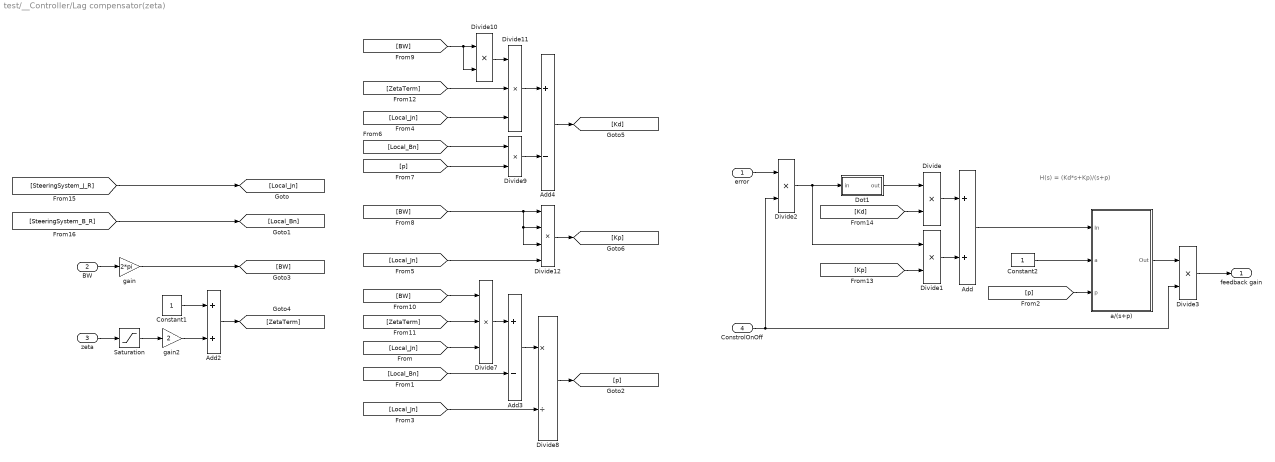
== system test/__Controller/Lag compensator(zeta) ==
  note: H(s) = (Kd*s+Kp)/(s+p)
  error : Inport
  BW : Inport  Port=2
  zeta : Inport  Port=3
  ConstrolOnOff : Inport  Port=4
  Add : Sum
  Add2 : Sum
  Add3 : Sum  Inputs=+-
  Add4 : Sum  Inputs=+-
  Constant1 : Constant  SampleTime=Ts
  Constant2 : Constant  SampleTime=Ts
  Divide{,1..3,9..10} (6 alike) : Product  Inputs=**
  Divide11 : Product  Inputs=***
  Divide12 : Product  Inputs=****
  Divide7 : Product  Inputs=***
  Divide8 : Product  Inputs=*/
  Dot1 : Subsystem
      mask Display: disp('dot')
  Saturation : Saturate  UpperLimit=1.5  LowerLimit=0.5
  a/(s+p) : Subsystem
  "gain " : Gain  Gain=2*pi
  gain2 : Gain  Gain=2
  feedback gain : Outport
  wires:
  BW/1 -> "gain "/1
  Add/1 -> a/(s+p)/1(In)
  Divide/1 -> Add/1
  Dot1/1(out) -> Divide/1
  Constant2/1 -> a/(s+p)/2(a)
  zeta/1 -> Saturation/1
  Saturation/1 -> gain2/1
  gain2/1 -> Add2/2
  Constant1/1 -> Add2/1
  [Local_Jn] -> Divide7/3
  Divide7/1 -> Add3/1
  [Local_Bn] -> Add3/2
  Add3/1 -> Divide8/1
  Divide10/1 -> Divide11/1
  Divide8/1 -> [p]
  Divide9/1 -> Add4/2
  Divide11/1 -> Add4/1
  [p] -> a/(s+p)/3(p)
  Divide1/1 -> Add/2
  [Local_Jn] -> Divide8/2
  [Local_Jn] -> Divide11/3
  [Local_Jn] -> Divide12/4
  [Local_Bn] -> Divide9/1
  [p] -> Divide9/2
  "gain "/1 -> [BW]
  [BW] -> Divide12/3, Divide12/2, Divide12/1
  [BW] -> Divide10/2, Divide10/1
  [BW] -> Divide7/1
  Add2/1 -> [ZetaTerm]
  [ZetaTerm] -> Divide7/2
  [ZetaTerm] -> Divide11/2
  Add4/1 -> [Kd]
  Divide12/1 -> [Kp]
  [Kp] -> Divide1/2
  [Kd] -> Divide/2
  [SteeringSystem_J_R] -> [Local_Jn]
  [SteeringSystem_B_R] -> [Local_Bn]
  error/1 -> Divide2/1
  Divide2/1 -> Divide1/1, Dot1/1(in)
  ConstrolOnOff/1 -> Divide3/2, Divide2/2
  a/(s+p)/1(Out) -> Divide3/1
  Divide3/1 -> feedback gain/1

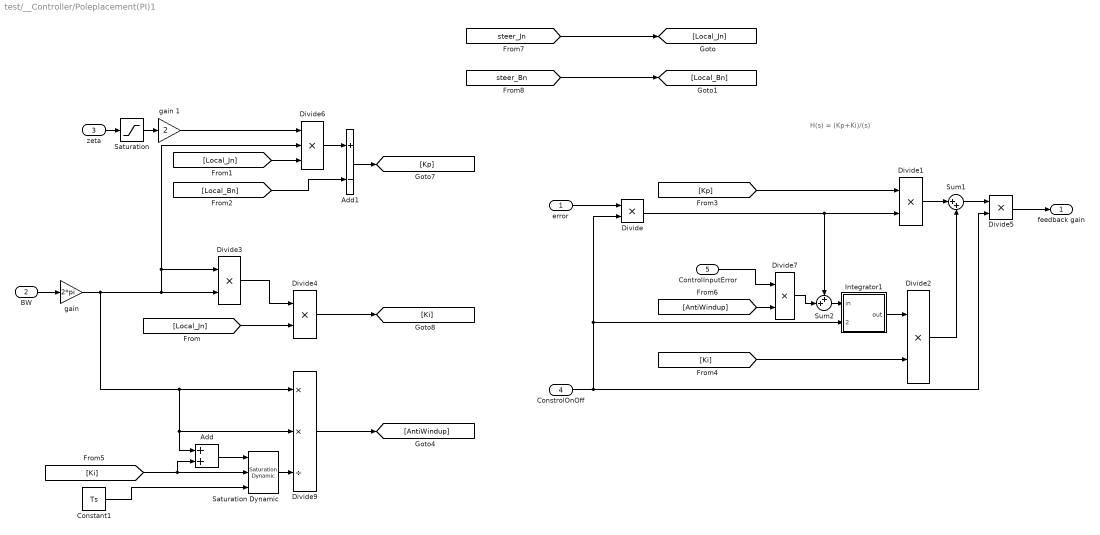
== system test/__Controller/Poleplacement(PI)1 ==
  note: H(s) = (Kp+Ki)/(s)
  error : Inport
  BW : Inport  Port=2
  zeta : Inport  Port=3
  ConstrolOnOff : Inport  Port=4
  ControlInputError : Inport  Port=5
  Add : Sum
  Add1 : Sum  Inputs=+-
  Constant1 : Constant  Value=Ts
  Divide{,1..5,7} (7 alike) : Product  Inputs=**
  Divide6 : Product  Inputs=***
  Divide9 : Product  Inputs=**/
  Integrator1 : Subsystem
      mask Display: disp('Integator')
  Saturation : Saturate  UpperLimit=3  LowerLimit=0.5
  Saturation Dynamic : simulink/Discontinuities/Saturation Dynamic  OutMin=[]  OutMax=[]  OutDataTypeStr=Inherit: Same as second input  OutDataType=fixdt(1, 16)  OutScaling=2^-10  DoSatur=off
  Sum1 : Sum  Inputs=|++
  Sum2 : Sum  Inputs=++|
  "gain " : Gain  Gain=2*pi
  gain 1 : Gain  Gain=2
  feedback gain : Outport
  wires:
  BW/1 -> "gain "/1
  zeta/1 -> Saturation/1
  Saturation/1 -> gain 1/1
  [Local_Bn] -> Add1/2
  Divide1/1 -> Sum1/1
  Divide2/1 -> Sum1/2
  Integrator1/1(out) -> Divide2/1
  gain 1/1 -> Divide6/1
  Divide3/1 -> Divide4/1
  [Local_Jn] -> Divide4/2
  [Local_Jn] -> Divide6/3
  Divide6/1 -> Add1/1
  Add1/1 -> [Kp]
  Divide4/1 -> [Ki]
  [Kp] -> Divide1/1
  error/1 -> Divide/1
  Sum1/1 -> Divide5/1
  Divide5/1 -> feedback gain/1
  ConstrolOnOff/1 -> Divide5/2, Integrator1/2("Off : 0 On : 1"), Divide/2
  [Ki] -> Divide2/2
  ControlInputError/1 -> Divide7/1
  Divide/1 -> Divide1/2, Sum2/1
  Sum2/1 -> Integrator1/1(in)
  Divide7/1 -> Sum2/2
  Add/1 -> Saturation Dynamic/1
  Divide9/1 -> [AntiWindup]
  Constant1/1 -> Saturation Dynamic/3
  "gain "/1 -> Divide9/2, Add/1, Divide9/1, Divide6/2, Divide3/1, Divide3/2
  [Ki] -> Add/2, Saturation Dynamic/2
  [AntiWindup] -> Divide7/2
  Saturation Dynamic/1 -> Divide9/3
  [steer_Jn] -> [Local_Jn]
  [steer_Bn] -> [Local_Bn]

== system test/__Controller/Steering system ==
  note: mN*m
  note: Motor N*m
  N*m : Inport
  Constant : Constant  Value=55.08
  Constant1 : Constant  Value=1000
  Constant2 : Constant
  Divide : Product  Inputs=*/
  Divide1 : Product  Inputs=**
  Divide3 : Product  Inputs=*/
  Gain : Gain  Gain=1000
  Gain1 : Gain  Gain=-1
  Saturation Dynamic : simulink/Discontinuities/Saturation Dynamic  OutMin=[]  OutMax=[]  OutDataTypeStr=Inherit: Same as second input  OutDataType=fixdt(1, 16)  OutScaling=2^-10  DoSatur=off
  Target Torque : Outport
  tag scope: closed_ID_FB=global
  wires:
  Constant2/1 -> Divide3/2
  Gain/1 -> Target Torque/1
  Divide/1 -> Gain/1
  N*m/1 -> Divide3/1
  Divide1/1 -> [closed_ID_FB], Saturation Dynamic/2
  Constant1/1 -> Divide1/2
  Divide3/1 -> Divide1/1
  Saturation Dynamic/1 -> Divide/1
  Gain1/1 -> Saturation Dynamic/3
  Constant/1 -> Saturation Dynamic/1, Gain1/1, Divide/2

== system test/__Controller/Subsystem1 ==
  note: wheel N*m
  note: mN*m
  note: Motor N*m
  N*m : Inport
  Constant : Constant  Value=55.08
  Constant1 : Constant  Value=1000
  Constant2 : Constant  Value=190
  Divide : Product  Inputs=*/
  Divide1 : Product  Inputs=**
  Divide3 : Product  Inputs=*/
  Gain : Gain  Gain=1000
  Gain1 : Gain  Gain=-1
  Saturation Dynamic : simulink/Discontinuities/Saturation Dynamic  OutMin=[]  OutMax=[]  OutDataTypeStr=Inherit: Same as second input  OutDataType=fixdt(1, 16)  OutScaling=2^-10  DoSatur=off
  Target Torque : Outport
  wires:
  Constant2/1 -> Divide3/2
  Gain/1 -> Target Torque/1
  Divide/1 -> Gain/1
  N*m/1 -> Divide3/1
  Divide1/1 -> Saturation Dynamic/2
  Constant1/1 -> Divide1/2
  Divide3/1 -> Divide1/1
  Saturation Dynamic/1 -> Divide/1
  Gain1/1 -> Saturation Dynamic/3
  Constant/1 -> Saturation Dynamic/1, Gain1/1, Divide/2

== system test/__Data Plotting/__Drive_Ctrl_Plot ==
  dri_ctrl_FF : Scope
  dri_ctrl_PID : Scope
  dri_ctrl_Total : Scope
  dri_ctrl_dhat : Scope
  wires:
  [dri_ctrl_dhat] -> dri_ctrl_dhat/1
  [dri_ctrl_Total] -> dri_ctrl_Total/1
  [dri_ctrl_FF] -> dri_ctrl_FF/1
  [dri_ctrl_PID] -> dri_ctrl_PID/1

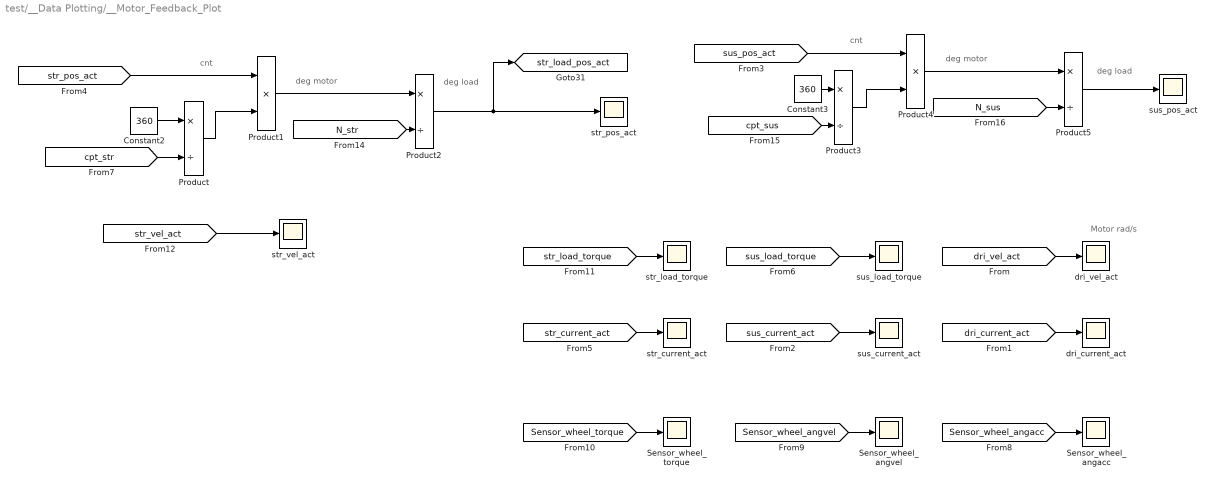
== system test/__Data Plotting/__Motor_Feedback_Plot ==
  note: Motor rad/s
  note: deg load
  note: cnt
  note: deg motor
  note: cnt
  note: deg motor
  note: deg load
  Constant2 : Constant  Value=360
  Constant3 : Constant  Value=360
  Product{,2..3,5} (4 alike) : Product  Inputs=*/
  Product1 : Product  Inputs=**
  Product4 : Product  Inputs=**
  Sensor_wheel_angacc : Scope
  Sensor_wheel_angvel : Scope
  Sensor_wheel_torque : Scope
  dri_current_act : Scope
  dri_vel_act : Scope
  str_current_act : Scope
  str_load_torque : Scope
  str_pos_act : Scope
  str_vel_act : Scope
  sus_current_act : Scope
  sus_load_torque : Scope
  sus_pos_act : Scope
  tag scope: str_load_pos_act=global
  wires:
  [str_current_act] -> str_current_act/1
  [Sensor_wheel_torque] -> Sensor_wheel_torque/1
  [Sensor_wheel_angvel] -> Sensor_wheel_angvel/1
  [dri_current_act] -> dri_current_act/1
  [dri_vel_act] -> dri_vel_act/1
  [sus_current_act] -> sus_current_act/1
  [Sensor_wheel_angacc] -> Sensor_wheel_angacc/1
  [str_load_torque] -> str_load_torque/1
  [sus_load_torque] -> sus_load_torque/1
  [str_pos_act] -> Product1/1
  [N_sus] -> Product5/2
  Product3/1 -> Product4/2
  Product4/1 -> Product5/1
  [sus_pos_act] -> Product4/1
  Product1/1 -> Product2/1
  Constant2/1 -> Product/1
  [cpt_sus] -> Product3/2
  Constant3/1 -> Product3/1
  Product5/1 -> sus_pos_act/1
  [N_str] -> Product2/2
  Product/1 -> Product1/2
  [cpt_str] -> Product/2
  [str_vel_act] -> str_vel_act/1
  Product2/1 -> [str_load_pos_act], str_pos_act/1

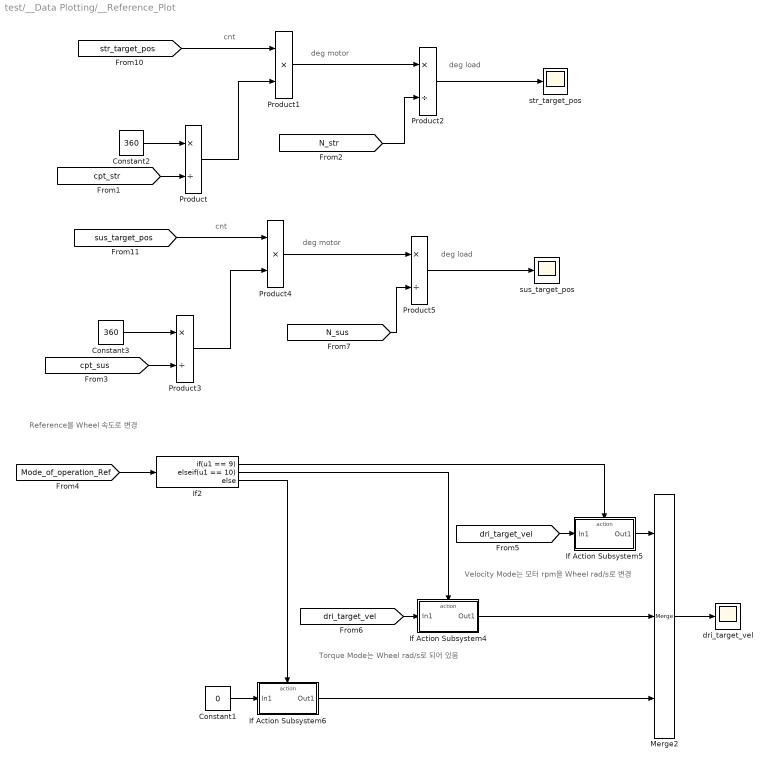
== system test/__Data Plotting/__Reference_Plot ==
  note: Torque Mode는 Wheel rad/s로 되어 있음
  note: Reference를 Wheel 속도로 변경
  note: Velocity Mode는 모터 rpm을 Wheel rad/s로 변경
  note: cnt
  note: deg motor
  note: deg load
  note: cnt
  note: deg motor
  note: deg load
  Constant1 : Constant  Value=0
  Constant2 : Constant  Value=360
  Constant3 : Constant  Value=360
  If Action Subsystem4 : Subsystem  TreatAsAtomicUnit=on
  If Action Subsystem5 : Subsystem  TreatAsAtomicUnit=on
  If Action Subsystem6 : Subsystem  TreatAsAtomicUnit=on
  If2 : If  IfExpression=u1 == 9  ElseIfExpressions=u1 == 10
  Merge2 : Merge  Inputs=3
  Product{,2..3,5} (4 alike) : Product  Inputs=*/
  Product1 : Product  Inputs=**
  Product4 : Product  Inputs=**
  dri_target_vel : Scope
  str_target_pos : Scope
  sus_target_pos : Scope
  wires:
  If2/2 -> If Action Subsystem4/Action
  If2/1 -> If Action Subsystem5/Action
  [dri_target_vel] -> If Action Subsystem5/1(In1)
  [Mode_of_operation_Ref] -> If2/1
  If2/3 -> If Action Subsystem6/Action
  Constant1/1 -> If Action Subsystem6/1(In1)
  If Action Subsystem4/1(Out1) -> Merge2/2
  If Action Subsystem6/1(Out1) -> Merge2/3
  [dri_target_vel] -> If Action Subsystem4/1(In1)
  If Action Subsystem5/1(Out1) -> Merge2/1
  Merge2/1 -> dri_target_vel/1
  Product/1 -> Product1/2
  Constant2/1 -> Product/1
  [str_target_pos] -> Product1/1
  Product2/1 -> str_target_pos/1
  Product1/1 -> Product2/1
  [cpt_str] -> Product/2
  [N_str] -> Product2/2
  [sus_target_pos] -> Product4/1
  Product5/1 -> sus_target_pos/1
  Product4/1 -> Product5/1
  [N_sus] -> Product5/2
  Product3/1 -> Product4/2
  [cpt_sus] -> Product3/2
  Constant3/1 -> Product3/1

== system test/__Data Plotting/__Sensor_Plot ==
  Acc_x : Scope
  Add : Sum  Inputs=+-
  Add1 : Sum  Inputs=+-
  Add2 : Sum  Inputs=+-
  Subsystem : Subsystem
      mask Display: disp('Vol2Newton')
  Subsystem1 : Subsystem
      mask Display: disp('Vol2Newton')
  grf_x : Scope
  grf_y : Scope
  wires:
  Subsystem/1(N) -> Add1/1
  [grf_y] -> Subsystem1/1(Voltage)
  [Acc_x] -> Add/1
  [Grf_x_bias] -> Add1/2
  Add2/1 -> grf_y/1
  Add1/1 -> grf_x/1
  [grf_x] -> Subsystem/1(Voltage)
  [Grf_y_bias] -> Add2/2
  Subsystem1/1(N) -> Add2/1
  [acc_bias] -> Add/2
  Add/1 -> Acc_x/1

== system test/__System_Setting/Subsystem ==
  In1 : Inport
  ID_Mode : Subsystem  TreatAsAtomicUnit=on
  If : If  IfExpression=u1 == 0  ElseIfExpressions=u1 == 1,u1 == 2
  Merge : Merge  Inputs=4
  Merge1 : Merge  Inputs=3
  Torque Mode : Subsystem  TreatAsAtomicUnit=on
  Torque Mode1 : Subsystem  TreatAsAtomicUnit=on
  Velocity Mode : Subsystem  TreatAsAtomicUnit=on
  tag scope: Driving_Ref_Mode=global, Mode_of_operation_Ref=global
  wires:
  In1/1 -> If/1
  If/1 -> Velocity Mode/Action
  If/2 -> Torque Mode/Action
  If/4 -> ID_Mode/Action
  Velocity Mode/1(Out1) -> Merge/1
  Torque Mode/1(Mode) -> Merge/2
  ID_Mode/1(Mode) -> Merge/3
  Merge/1 -> [Mode_of_operation_Ref]
  Torque Mode/2(Out2) -> Merge1/1
  ID_Mode/2(Out2) -> Merge1/3
  Merge1/1 -> [Driving_Ref_Mode]
  If/3 -> Torque Mode1/Action
  Torque Mode1/2(Out2) -> Merge1/2
  Torque Mode1/1(Mode) -> Merge/4

== system test/RTI Data/RTI Data Store/RTI Data Store ==
  RTI Data Store : Subsystem  mask(RTI_DATA_STORE){}
      mask help:
      | RTI Data Store Block. This block is used by RTI to store internal model dependent data. Deleting this block will result in data loss.
      |
      | NEVER DELETE, COPY, OR MODIFY THIS BLOCK!
      mask Help:
      | RTI Data Store Block. This block is used by RTI to store internal model dependent data. Deleting this block will result in data loss.
      | 
      | NEVER DELETE, COPY, OR MODIFY THIS BLOCK!
      mask Display: text(0.5, 0.5, ' ', 'HorizontalAlignment', 'center');

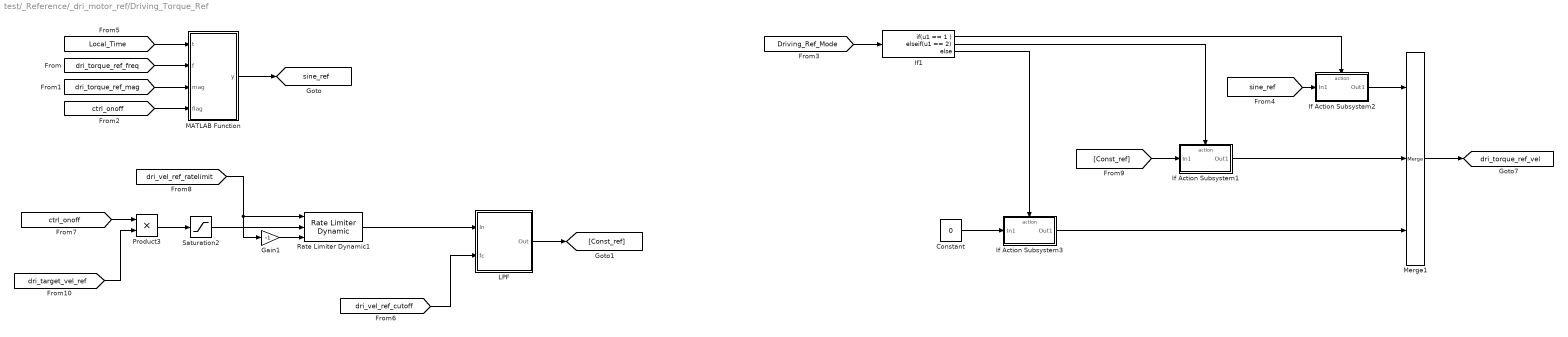
== system test/_Reference/_dri_motor_ref/Driving_Torque_Ref ==
  Constant : Constant  Value=0
  Gain1 : Gain  Gain=-1
  If Action Subsystem1 : Subsystem  TreatAsAtomicUnit=on
  If Action Subsystem2 : Subsystem  TreatAsAtomicUnit=on
  If Action Subsystem3 : Subsystem  TreatAsAtomicUnit=on
  If1 : If  IfExpression=u1 == 1  ElseIfExpressions=u1 == 2
  LPF : Subsystem
  MATLAB Function : MATLAB Function  TreatAsAtomicUnit=on
  Merge1 : Merge  Inputs=3
  Product3 : Product
  Rate Limiter Dynamic1 : simulink/Discontinuities/Rate Limiter Dynamic
      settings: SourceProductName=Simulink
  Saturation2 : Saturate  UpperLimit=10  LowerLimit=-10
  tag scope: dri_torque_ref_vel=global, sine_ref=global
  wires:
  [Local_Time] -> MATLAB Function/1(t)
  MATLAB Function/1(y) -> [sine_ref]
  [dri_torque_ref_freq] -> MATLAB Function/2(f)
  [dri_torque_ref_mag] -> MATLAB Function/3(mag)
  [ctrl_onoff] -> MATLAB Function/4(flag)
  Merge1/1 -> [dri_torque_ref_vel]
  [Driving_Ref_Mode] -> If1/1
  If1/1 -> If Action Subsystem2/Action
  Gain1/1 -> Rate Limiter Dynamic1/3
  Product3/1 -> Saturation2/1
  [dri_target_vel_ref] -> Product3/2
  [dri_vel_ref_ratelimit] -> Rate Limiter Dynamic1/1, Gain1/1
  Rate Limiter Dynamic1/1 -> LPF/1(In)
  [dri_vel_ref_cutoff] -> LPF/2(fc)
  [ctrl_onoff] -> Product3/1
  Saturation2/1 -> Rate Limiter Dynamic1/2
  [sine_ref] -> If Action Subsystem2/1(In1)
  If Action Subsystem2/1(Out1) -> Merge1/1
  LPF/1(Out) -> [Const_ref]
  [Const_ref] -> If Action Subsystem1/1(In1)
  If1/2 -> If Action Subsystem1/Action
  If Action Subsystem1/1(Out1) -> Merge1/2
  If Action Subsystem3/1(Out1) -> Merge1/3
  If1/3 -> If Action Subsystem3/Action
  Constant/1 -> If Action Subsystem3/1(In1)

== system test/_Reference/_dri_motor_ref/Driving_Vel_Ref ==
  note: m/s
  note: Wheel deg/s
  note: Motor deg/s
  note: RPM
  Constant2 : Constant  Value=2*pi
  Constant3 : Constant  Value=360
  Constant4 : Constant  Value=60/360
  Data Type Conversion2 : DataTypeConversion
  Gain1 : Gain  Gain=-1
  LPF : Subsystem
  Product{3,6..8,10} (5 alike) : Product
  Product9 : Product  Inputs=*/
  Rate Limiter Dynamic1 : simulink/Discontinuities/Rate Limiter Dynamic
      settings: SourceProductName=Simulink
  Saturation2 : Saturate  UpperLimit=10  LowerLimit=-10
  tag scope: dri_velocity_ref_vel=global
  wires:
  Product6/1 -> Product7/1
  Constant2/1 -> Product8/1
  [dri_vel_ref_cutoff] -> LPF/2(fc)
  [N_dri] -> Product7/2
  Saturation2/1 -> Rate Limiter Dynamic1/2
  Constant4/1 -> Product10/2
  LPF/1(Out) -> Product6/1
  Product9/1 -> Product6/2
  Constant3/1 -> Product9/1
  Product8/1 -> Product9/2
  Rate Limiter Dynamic1/1 -> LPF/1(In)
  Product7/1 -> Product10/1
  Product10/1 -> Data Type Conversion2/1
  [radius] -> Product8/2
  [ctrl_onoff] -> Product3/1
  [dri_target_vel_ref] -> Product3/2
  Gain1/1 -> Rate Limiter Dynamic1/3
  Product3/1 -> Saturation2/1
  Data Type Conversion2/1 -> [dri_velocity_ref_vel]
  [dri_vel_ref_ratelimit] -> Rate Limiter Dynamic1/1, Gain1/1

== system test/_Reference/_dri_motor_ref/If Action Subsystem1 ==
  In1 : Inport
  Action Port : ActionPort  ActionType=elseif
  Out1 : Outport
  wires:
  In1/1 -> Out1/1

== system test/_Reference/_dri_motor_ref/If Action Subsystem2 ==
  In1 : Inport
  Action Port : ActionPort  ActionType=then
  Out1 : Outport
  wires:
  In1/1 -> Out1/1

== system test/_Reference/_dri_motor_ref/If Action Subsystem3 ==
  In1 : Inport
  Action Port : ActionPort  ActionType=else
  Out1 : Outport
  wires:
  In1/1 -> Out1/1
